simulink model "jk"  (R2018a)
settings: Solver=FixedStepDiscrete  StartTime=0.0  StopTime=10.0  FixedStep=10e-6  RelTol=1e-3
libraries: neural x37, powerlib x17, simulink x1, re_lib x1, powerlib_meascontrol x1
(part 2 of 2)

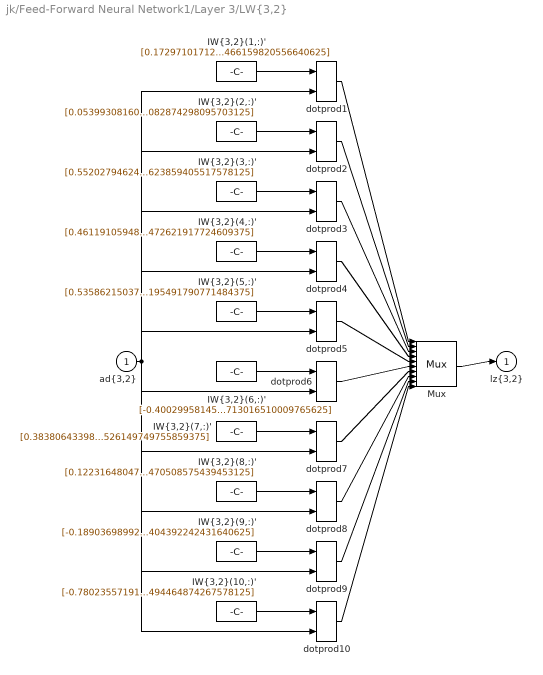
== system jk/Feed-Forward Neural Network1/Layer 3/LW{3,2} ==
  "ad{3,2}" : Inport  PortDimensions=10
      mask Display: e = 0.06;c1 = [120 230 180]/255;c2 = ([120 230 180]+0)/(256+128);c3 = ([120 230 180]+128)/(256+128);patch([0 1 1 0],[0 0 1 1],c1);patch([0 1 1 1-e 1-e 0+e],[0 0 1 1-e 0+e 0+e],c2);patch([0 0 1 1-e 0+e 0+e],[0 1 1 1-e 1-e 0+e],c3);plot([0 1 1 0 0],[0 0 1 1 0]);
  "IW{3,2}(1,:)'" : Constant  Value=[0.17297101712737783518747392008663155138492584228515625;0.478025722941598452120359752370859496295452117919921875;0.403245851675728184115854446645244024693965911865234375;-0.66539393369935506683532366878353059291839599609375;0.63017645254385701303334599288064055144786834716796875;0.465121336368979620967678556553437374532222747802734375;-0.363851749702136129105412010176223702728748321533203125;0.80326730275410318515838525854633189737796783447265625;0.50830526031887035554035492168623022735118865966796875;-0.76780955124176986092976449072011746466159820556640625]
      mask Display: e = 0.06;c1 = [120 150 230]/255;c2 = ([120 150 230]+0)/383;c3 = ([120 150 230]+128)/383;patch([0 1 1 0],[0 0 1 1],c1);patch([0 1 1 1-e 1-e 0+e],[0 0 1 1-e 0+e 0+e],c2);patch([0 0 1 1-e 0+e 0+e],[0 1 1 1-e 1-e 0+e],c3);plot([0 1 1 0 0],[0 0 1 1 0]);disp('weights');
  "IW{3,2}(10,:)'" : Constant  Value=[-0.78023557191233539054309176208334974944591522216796875;0.4761460635207281910652454826049506664276123046875;-0.6823292834328154032874635959160514175891876220703125;0.76798052215580747681400453075184486806392669677734375;-0.693161939288044148810286060324870049953460693359375;-0.627626419206150476526318016112782061100006103515625;0.1181635050366092176687971004866994917392730712890625;-0.37675514077040095362036709047970362007617950439453125;0.1557106833714762272879994497998268343508243560791015625;0.2231410893052308275219530742106144316494464874267578125]
      mask Display: e = 0.06;c1 = [120 150 230]/255;c2 = ([120 150 230]+0)/383;c3 = ([120 150 230]+128)/383;patch([0 1 1 0],[0 0 1 1],c1);patch([0 1 1 1-e 1-e 0+e],[0 0 1 1-e 0+e 0+e],c2);patch([0 0 1 1-e 0+e 0+e],[0 1 1 1-e 1-e 0+e],c3);plot([0 1 1 0 0],[0 0 1 1 0]);disp('weights');
  "IW{3,2}(2,:)'" : Constant  Value=[0.053993081609670139087153728496559779159724712371826171875;-0.347860530824692426588029547929181717336177825927734375;-0.9976428845241078757766217677271924912929534912109375;0.311012259102058374882204816458397544920444488525390625;-0.95037076652526575326618285544100217521190643310546875;-0.63681687252203145188644839436165057122707366943359375;-0.60370147389502337720301738954731263220310211181640625;-0.1267767660075609370551319443620741367340087890625;-0.05310864953495571250119411388368462212383747100830078125;-0.421912552543257046711033808605861850082874298095703125]
      mask Display: e = 0.06;c1 = [120 150 230]/255;c2 = ([120 150 230]+0)/383;c3 = ([120 150 230]+128)/383;patch([0 1 1 0],[0 0 1 1],c1);patch([0 1 1 1-e 1-e 0+e],[0 0 1 1-e 0+e 0+e],c2);patch([0 0 1 1-e 0+e 0+e],[0 1 1 1-e 1-e 0+e],c3);plot([0 1 1 0 0],[0 0 1 1 0]);disp('weights');
  "IW{3,2}(3,:)'" : Constant  Value=[0.5520279462491097799414774272008799016475677490234375;0.1648188595326314509481591130679589696228504180908203125;-1.04652829460949892137477945652790367603302001953125;-0.47402449147789693650878461994579993188381195068359375;-0.277885579664090887064276103046722710132598876953125;-0.2201686272549187306513118755901814438402652740478515625;-0.01485216057259106277321780709144150023348629474639892578125;0.476205043403078231989411506219767034053802490234375;0.74952531985042336604152524159871973097324371337890625;0.66261370244167938636792314355261623859405517578125]
      mask Display: e = 0.06;c1 = [120 150 230]/255;c2 = ([120 150 230]+0)/383;c3 = ([120 150 230]+128)/383;patch([0 1 1 0],[0 0 1 1],c1);patch([0 1 1 1-e 1-e 0+e],[0 0 1 1-e 0+e 0+e],c2);patch([0 0 1 1-e 0+e 0+e],[0 1 1 1-e 1-e 0+e],c3);plot([0 1 1 0 0],[0 0 1 1 0]);disp('weights');
  "IW{3,2}(4,:)'" : Constant  Value=[0.461191059485868082301607273620902560651302337646484375;0.54161132101339826139252409120672382414340972900390625;-0.9231210633499602469242972802021540701389312744140625;0.3338185036025709262474947536247782409191131591796875;-0.304789913565141734608232582104392349720001220703125;0.09868186364481952577154544314907980151474475860595703125;-0.9148409326736413049729890190064907073974609375;0.5906418231625283343788623824366368353366851806640625;-0.252691266444447837358211472746916115283966064453125;0.4359690288000626079423227565712295472621917724609375]
      mask Display: e = 0.06;c1 = [120 150 230]/255;c2 = ([120 150 230]+0)/383;c3 = ([120 150 230]+128)/383;patch([0 1 1 0],[0 0 1 1],c1);patch([0 1 1 1-e 1-e 0+e],[0 0 1 1-e 0+e 0+e],c2);patch([0 0 1 1-e 0+e 0+e],[0 1 1 1-e 1-e 0+e],c3);plot([0 1 1 0 0],[0 0 1 1 0]);disp('weights');
  "IW{3,2}(5,:)'" : Constant  Value=[0.5358621503719811496324609834118746221065521240234375;-0.89157502449929493248959033735445700585842132568359375;0.6351119924327439658640059860772453248500823974609375;0.47178887457483165146499004549696110188961029052734375;0.41226330362267094020722879577078856527805328369140625;-0.5120710986545276011128180471132509410381317138671875;-0.310488497392649109851703315143822692334651947021484375;-0.12352606296812708441823502880652085877954959869384765625;-0.4909360423967399356115492992103099822998046875;-0.84133587929376874026132782091735862195491790771484375]
      mask Display: e = 0.06;c1 = [120 150 230]/255;c2 = ([120 150 230]+0)/383;c3 = ([120 150 230]+128)/383;patch([0 1 1 0],[0 0 1 1],c1);patch([0 1 1 1-e 1-e 0+e],[0 0 1 1-e 0+e 0+e],c2);patch([0 0 1 1-e 0+e 0+e],[0 1 1 1-e 1-e 0+e],c3);plot([0 1 1 0 0],[0 0 1 1 0]);disp('weights');
  "IW{3,2}(6,:)'" : Constant  Value=[-0.400299581456519171229757603214238770306110382080078125;-0.6905620981717308648484277000534348189830780029296875;0.81990341779897402130217187732341699302196502685546875;0.13412505817003783636920388744329102337360382080078125;0.202530670147044011830672616270021535456180572509765625;0.233224627115440175106897413570550270378589630126953125;-0.71505424960624852648294336177059449255466461181640625;0.2566456114750599315499357544467784464359283447265625;-0.82212921393638271894133140449412167072296142578125;-0.683689673205540859868278857902623713016510009765625]
      mask Display: e = 0.06;c1 = [120 150 230]/255;c2 = ([120 150 230]+0)/383;c3 = ([120 150 230]+128)/383;patch([0 1 1 0],[0 0 1 1],c1);patch([0 1 1 1-e 1-e 0+e],[0 0 1 1-e 0+e 0+e],c2);patch([0 0 1 1-e 0+e 0+e],[0 1 1 1-e 1-e 0+e],c3);plot([0 1 1 0 0],[0 0 1 1 0]);disp('weights');
  "IW{3,2}(7,:)'" : Constant  Value=[0.383806433989951234497794985145446844398975372314453125;0.045518664553806827133275447749838349409401416778564453125;0.38302565829951940035158486352884210646152496337890625;0.49567557860381461498633370865718461573123931884765625;0.71373012188424789226104394401772879064083099365234375;0.0229740235719602496622382403757001156918704509735107421875;-0.739517436109949688471942863543517887592315673828125;-0.76512701135517235950800341015565209090709686279296875;0.388353426727468475920801438405760563910007476806640625;-0.86727676170474621297756812055013142526149749755859375]
      mask Display: e = 0.06;c1 = [120 150 230]/255;c2 = ([120 150 230]+0)/383;c3 = ([120 150 230]+128)/383;patch([0 1 1 0],[0 0 1 1],c1);patch([0 1 1 1-e 1-e 0+e],[0 0 1 1-e 0+e 0+e],c2);patch([0 0 1 1-e 0+e 0+e],[0 1 1 1-e 1-e 0+e],c3);plot([0 1 1 0 0],[0 0 1 1 0]);disp('weights');
  "IW{3,2}(8,:)'" : Constant  Value=[0.12231648047044048344123012839190778322517871856689453125;-0.10546690293607696720101785103906877338886260986328125;-0.73134552615097014882650228173588402569293975830078125;-0.50796732023131785371816704355296678841114044189453125;-0.19051910429759899567869751990656368434429168701171875;-0.55906816359749200717743633504142053425312042236328125;0.5331202300770805369012350638513453304767608642578125;0.85261855049123502769958804492489434778690338134765625;-0.06722752675672520605854032282877597026526927947998046875;-0.918475872125970926873606003937311470508575439453125]
      mask Display: e = 0.06;c1 = [120 150 230]/255;c2 = ([120 150 230]+0)/383;c3 = ([120 150 230]+128)/383;patch([0 1 1 0],[0 0 1 1],c1);patch([0 1 1 1-e 1-e 0+e],[0 0 1 1-e 0+e 0+e],c2);patch([0 0 1 1-e 0+e 0+e],[0 1 1 1-e 1-e 0+e],c3);plot([0 1 1 0 0],[0 0 1 1 0]);disp('weights');
  "IW{3,2}(9,:)'" : Constant  Value=[-0.189036989924661169570896390723646618425846099853515625;0.95016371798828214156884541807812638580799102783203125;0.501473757210082471402756709721870720386505126953125;0.63135497163872245085514123275061137974262237548828125;-0.56201031605421281067691552379983477294445037841796875;0.65029748784733631961074706850922666490077972412109375;-0.398730903333880559724633485529921017587184906005859375;-0.80631825806199952655362039877218194305896759033203125;0.005402005041339444542380920921686993096955120563507080078125;-0.113738532944788917067313605002709664404392242431640625]
      mask Display: e = 0.06;c1 = [120 150 230]/255;c2 = ([120 150 230]+0)/383;c3 = ([120 150 230]+128)/383;patch([0 1 1 0],[0 0 1 1],c1);patch([0 1 1 1-e 1-e 0+e],[0 0 1 1-e 0+e 0+e],c2);patch([0 0 1 1-e 0+e 0+e],[0 1 1 1-e 1-e 0+e],c3);plot([0 1 1 0 0],[0 0 1 1 0]);disp('weights');
  Mux : Mux  Inputs=10
      mask Display: e = 0.06;c1 = [120 150 230]/255;c2 = ([120 150 230]+0)/383;c3 = ([120 150 230]+128)/383;patch([0 1 1 0],[0 0 1 1],c1);patch([0 1 1 1-e 1-e 0+e],[0 0 1 1-e 0+e 0+e],c2);patch([0 0 1 1-e 0+e 0+e],[0 1 1 1-e 1-e 0+e],c3);plot([0 1 1 0 0],[0 0 1 1 0]);disp('Mux');
  dotprod{1..10} (10 alike) : neural/Weight Functions/dotprod
  "lz{3,2}" : Outport
      mask Display: e = 0.06;c1 = [120 230 180]/255;c2 = ([120 230 180]+0)/(256+128);c3 = ([120 230 180]+128)/(256+128);patch([0 1 1 0],[0 0 1 1],c1);patch([0 1 1 1-e 1-e 0+e],[0 0 1 1-e 0+e 0+e],c2);patch([0 0 1 1-e 0+e 0+e],[0 1 1 1-e 1-e 0+e],c3);plot([0 1 1 0 0],[0 0 1 1 0]);
  wires:
  "IW{3,2}(1,:)'"/1 -> dotprod1/1
  "ad{3,2}"/1 -> dotprod1/2, dotprod2/2, dotprod3/2, dotprod4/2, dotprod5/2, dotprod6/2, dotprod7/2, dotprod8/2, dotprod9/2, dotprod10/2
  dotprod1/1 -> Mux/1
  "IW{3,2}(2,:)'"/1 -> dotprod2/1
  dotprod2/1 -> Mux/2
  "IW{3,2}(3,:)'"/1 -> dotprod3/1
  dotprod3/1 -> Mux/3
  "IW{3,2}(4,:)'"/1 -> dotprod4/1
  dotprod4/1 -> Mux/4
  "IW{3,2}(5,:)'"/1 -> dotprod5/1
  dotprod5/1 -> Mux/5
  "IW{3,2}(6,:)'"/1 -> dotprod6/1
  dotprod6/1 -> Mux/6
  "IW{3,2}(7,:)'"/1 -> dotprod7/1
  dotprod7/1 -> Mux/7
  "IW{3,2}(8,:)'"/1 -> dotprod8/1
  dotprod8/1 -> Mux/8
  "IW{3,2}(9,:)'"/1 -> dotprod9/1
  dotprod9/1 -> Mux/9
  "IW{3,2}(10,:)'"/1 -> dotprod10/1
  dotprod10/1 -> Mux/10
  Mux/1 -> "lz{3,2}"/1

== system jk/Feed-Forward Neural Network1/Layer 4/Delays 1 ==
  "p{4}" : Inport  PortDimensions=10
      mask Display: e = 0.06;c1 = [120 230 180]/255;c2 = ([120 230 180]+0)/(256+128);c3 = ([120 230 180]+128)/(256+128);patch([0 1 1 0],[0 0 1 1],c1);patch([0 1 1 1-e 1-e 0+e],[0 0 1 1-e 0+e 0+e],c2);patch([0 0 1 1-e 0+e 0+e],[0 1 1 1-e 1-e 0+e],c3);plot([0 1 1 0 0],[0 0 1 1 0]);
  mux : Mux  Inputs=1
      mask Display: e = 0.06;c1 = [120 150 230]/255;c2 = ([120 150 230]+0)/383;c3 = ([120 150 230]+128)/383;patch([0 1 1 0],[0 0 1 1],c1);patch([0 1 1 1-e 1-e 0+e],[0 0 1 1-e 0+e 0+e],c2);patch([0 0 1 1-e 0+e 0+e],[0 1 1 1-e 1-e 0+e],c3);plot([0 1 1 0 0],[0 0 1 1 0]);disp('Mux')
  "pd{4,3}" : Outport
      mask Display: e = 0.06;c1 = [120 230 180]/255;c2 = ([120 230 180]+0)/(256+128);c3 = ([120 230 180]+128)/(256+128);patch([0 1 1 0],[0 0 1 1],c1);patch([0 1 1 1-e 1-e 0+e],[0 0 1 1-e 0+e 0+e],c2);patch([0 0 1 1-e 0+e 0+e],[0 1 1 1-e 1-e 0+e],c3);plot([0 1 1 0 0],[0 0 1 1 0]);
  wires:
  "p{4}"/1 -> mux/1
  mux/1 -> "pd{4,3}"/1

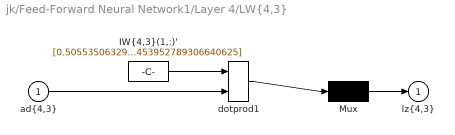
== system jk/Feed-Forward Neural Network1/Layer 4/LW{4,3} ==
  "ad{4,3}" : Inport  PortDimensions=10
      mask Display: e = 0.06;c1 = [120 230 180]/255;c2 = ([120 230 180]+0)/(256+128);c3 = ([120 230 180]+128)/(256+128);patch([0 1 1 0],[0 0 1 1],c1);patch([0 1 1 1-e 1-e 0+e],[0 0 1 1-e 0+e 0+e],c2);patch([0 0 1 1-e 0+e 0+e],[0 1 1 1-e 1-e 0+e],c3);plot([0 1 1 0 0],[0 0 1 1 0]);
  "IW{4,3}(1,:)'" : Constant  Value=[0.50553506329619946058073765016160905361175537109375;0.0948696855161368091113871514608035795390605926513671875;-0.7718944279241186645634797969250939786434173583984375;0.1003262319830757476335492128782789222896099090576171875;-0.78839627638930986908150089220725931227207183837890625;-0.6508990133213818918278548153466545045375823974609375;-0.92876201210975850575124468377907760441303253173828125;-0.51588785062832409611388584380620159208774566650390625;-0.5101977551512237862851861791568808257579803466796875;-0.4984173072461575149105783566483296453952789306640625]
      mask Display: e = 0.06;c1 = [120 150 230]/255;c2 = ([120 150 230]+0)/383;c3 = ([120 150 230]+128)/383;patch([0 1 1 0],[0 0 1 1],c1);patch([0 1 1 1-e 1-e 0+e],[0 0 1 1-e 0+e 0+e],c2);patch([0 0 1 1-e 0+e 0+e],[0 1 1 1-e 1-e 0+e],c3);plot([0 1 1 0 0],[0 0 1 1 0]);disp('weights');
  Mux : Mux  Inputs=1
      mask Display: e = 0.06;c1 = [120 150 230]/255;c2 = ([120 150 230]+0)/383;c3 = ([120 150 230]+128)/383;patch([0 1 1 0],[0 0 1 1],c1);patch([0 1 1 1-e 1-e 0+e],[0 0 1 1-e 0+e 0+e],c2);patch([0 0 1 1-e 0+e 0+e],[0 1 1 1-e 1-e 0+e],c3);plot([0 1 1 0 0],[0 0 1 1 0]);disp('Mux');
  dotprod1 : neural/Weight Functions/dotprod
  "lz{4,3}" : Outport
      mask Display: e = 0.06;c1 = [120 230 180]/255;c2 = ([120 230 180]+0)/(256+128);c3 = ([120 230 180]+128)/(256+128);patch([0 1 1 0],[0 0 1 1],c1);patch([0 1 1 1-e 1-e 0+e],[0 0 1 1-e 0+e 0+e],c2);patch([0 0 1 1-e 0+e 0+e],[0 1 1 1-e 1-e 0+e],c3);plot([0 1 1 0 0],[0 0 1 1 0]);
  wires:
  "IW{4,3}(1,:)'"/1 -> dotprod1/1
  "ad{4,3}"/1 -> dotprod1/2
  dotprod1/1 -> Mux/1
  Mux/1 -> "lz{4,3}"/1
